simulink model "ampc_pH_lmpc"  (R2021a)
settings: Solver=VariableStepAuto  StartTime=0.0  StopTime=400  RelTol=1e-3
undefined symbols (not defined in the file or in its folder): sigbuilder_block
libraries: mpclib x1, simulink x1
settings Model: Creator=USER  LastModifiedBy=USER

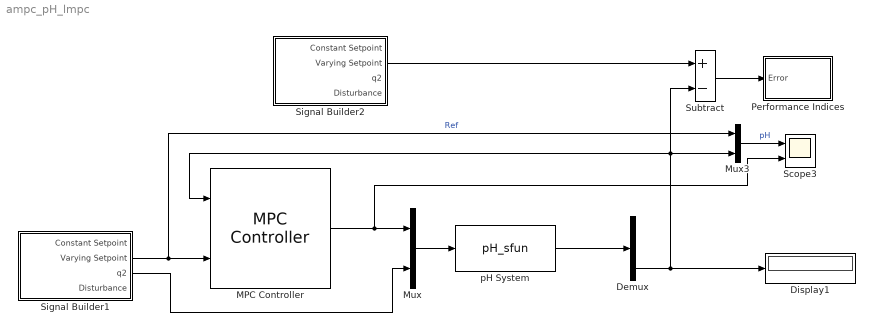
== system ampc_pH_lmpc ==
  Demux : Demux  Outputs=3
  Display1 : Display
  MPC Controller : mpclib/MPC Controller  SCDEnableBlockLinearizationSpecification=on  mpcobj=mpcobj_lmpc  is_multiple=0  enable_value=0  return_u0=off  updateMPCinCallerWorkspace=on  md_inport=off  mv_inport=off  uref_inport=off  return_cost=off  return_mvseq=off  return_qpstatus=off  return_xseq=off  return_state=off  return_ovseq=off  state_inport=off  umin_inport=off  umax_inport=off  ymin_inport=off  ymax_inport=off  cc_inport=off  ywt_inport=off  uwt_inport=off  duwt_inport=off  rhoeps_inport=off  pm_inport=off  MaximumP=10  HorizonChoice=FixedHorizon  n_ts=0.5  n_p=20  n_mv=1  n_md=0  n_ud=0  n_mo=1  n_uo=0  BlockDataType=double  SampleTimeInherited=off  switch_inport=off
  Mux : Mux  Inputs=2
  Mux3 : Mux  Inputs=2
  Performance Indices : Subsystem
  Scope3 : Scope  NumInputPorts=2
  Signal Builder1 : Subsystem  Tag=STV Subsys  LoadFcn=sigbuilder_block('load');  StartFcn=sigbuilder_block('start');  StopFcn=sigbuilder_block('stop');  ClipboardFcn=sigbuilder_block('clipboard');  mask(Sigbuilder block){tuvar=[0:10]}
      mask help: Simulink:masks:SigbuilderBlock_MD
      mask init:
      | if ~strcmp(get_param(bdroot(gcbh),'SimulationStatus'),'stopped') tuvar = sigbuilder_block('maskInit'); end
      settings: CopyFcn=sigbuilder_block('copy');  DeleteFcn=sigbuilder_block('delete');  ModelCloseFcn=sigbuilder_block('modelClose');  PreSaveFcn=sigbuilder_block('preSave');  PauseFcn=sigbuilder_block('pause');  ContinueFcn=sigbuilder_block('continue');  NameChangeFcn=sigbuilder_block('namechange');  OpenFcn=sigbuilder_block('open',[301 130.5 653.5 349.5 ]);  CloseFcn=sigbuilder_block('close');
      mask Display: plot(0, 0, 100, 100,[2, 2, 32, 32, 2], [68, 8, 8, 68, 68],[32, 2], [38, 38], [32, 19, 2],[53, 60, 44], [32, 17, 17, 2],[16, 16, 31, 31]);txt = getActiveGroup(gcbh);text(2, 100, txt,'verticalAlignment', 'top');
  Signal Builder2 : Subsystem  Tag=STV Subsys  LoadFcn=sigbuilder_block('load');  StartFcn=sigbuilder_block('start');  StopFcn=sigbuilder_block('stop');  ClipboardFcn=sigbuilder_block('clipboard');  mask(Sigbuilder block){tuvar=[0:10]}
      mask help: Simulink:masks:SigbuilderBlock_MD
      mask init:
      | if ~strcmp(get_param(bdroot(gcbh),'SimulationStatus'),'stopped') tuvar = sigbuilder_block('maskInit'); end
      settings: CopyFcn=sigbuilder_block('copy');  DeleteFcn=sigbuilder_block('delete');  ModelCloseFcn=sigbuilder_block('modelClose');  PreSaveFcn=sigbuilder_block('preSave');  PauseFcn=sigbuilder_block('pause');  ContinueFcn=sigbuilder_block('continue');  NameChangeFcn=sigbuilder_block('namechange');  OpenFcn=sigbuilder_block('open',[301 130.5 653.5 349.5 ]);  CloseFcn=sigbuilder_block('close');
      mask Display: plot(0, 0, 100, 100,[2, 2, 32, 32, 2], [68, 8, 8, 68, 68],[32, 2], [38, 38], [32, 19, 2],[53, 60, 44], [32, 17, 17, 2],[16, 16, 31, 31]);txt = getActiveGroup(gcbh);text(2, 100, txt,'verticalAlignment', 'top');
  Subtract : Sum  Inputs=+-
  pH System : S-Function  FunctionName=pH_sfun  SFunctionDeploymentMode=off  EnableBusSupport=off
  wires:
  Signal Builder1/2(Varying Setpoint) -> Mux3/1, MPC Controller/2  "Ref"
  Mux3/1 -> Scope3/1  "pH"
  Signal Builder2/2(Varying Setpoint) -> Subtract/1
  Subtract/1 -> Performance Indices/1(Error)
  MPC Controller/1 -> Scope3/2, Mux/1
  Signal Builder1/3(q2) -> Mux/2
  Demux/3 -> Display1/1, MPC Controller/1, Subtract/2, Mux3/2
  pH System/1 -> Demux/1
  Mux/1 -> pH System/1

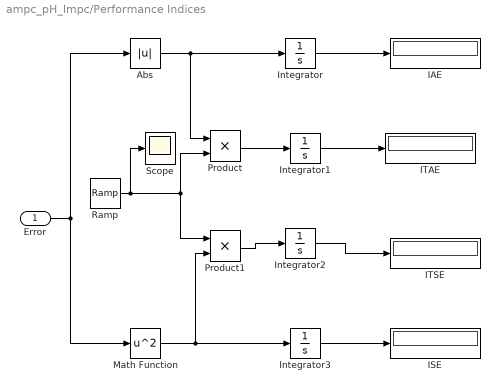
== system ampc_pH_lmpc/Performance Indices ==
  Error : Inport
  Abs : Abs
  IAE : Display
  ISE : Display
  ITAE : Display
  ITSE : Display
  Integrator{,1..3} (4 alike) : Integrator
  Math Function : Math  Operator=square  SignedPower=on  SaturateOnIntegerOverflow=on
  Product : Product  RndMeth=Zero
  Product1 : Product  RndMeth=Zero
  Ramp : simulink/Sources/Ramp  slope=1  start=0  InitialOutput=0
  Scope : Scope
  wires:
  Error/1 -> Math Function/1, Abs/1
  Abs/1 -> Integrator/1, Product/1
  Integrator/1 -> IAE/1
  Ramp/1 -> Product/2, Product1/1, Scope/1
  Math Function/1 -> Integrator3/1, Product1/2
  Product1/1 -> Integrator2/1
  Product/1 -> Integrator1/1
  Integrator3/1 -> ISE/1
  Integrator2/1 -> ITSE/1
  Integrator1/1 -> ITAE/1

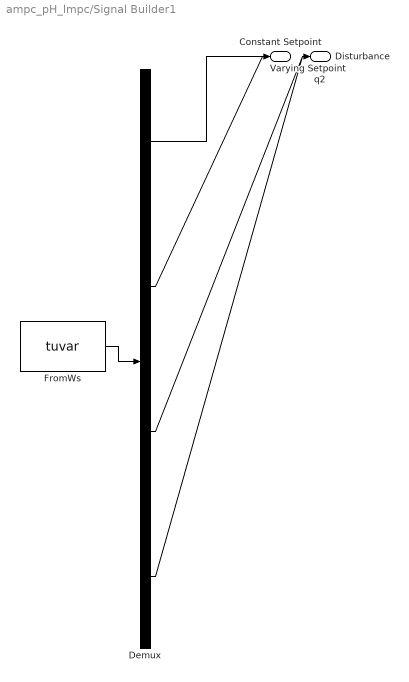
== system ampc_pH_lmpc/Signal Builder1 ==
  Demux : Demux  Tag=STV Demux
      settings: DisplayOption=none
  FromWs : FromWorkspace  Tag=STV FromWs  VariableName=tuvar
      SigBuilderData=|
      | common.afterFinalStr = 'Extrapolate'
      | common.sampleTime = 0
      | dataSet(1).timeRange = [0 400]
      | dataSet(1).name = 'Servo'
      | dataSet(2).timeRange = [0 400]
      | dataSet(2).name = 'Regulatory'
      | sbobj.Groups(1).Name = 'Servo'
      | sbobj.Groups(1).Signals(1).Name = 'Constant Setpoint'
      | sbobj.Groups(1).Signals(1).XData = [0 400]
      | sbobj.Groups(1).Signals(1).YData = [7 7]
      | sbobj.Groups(1).Signals(2).Name = 'Varying Setpoint'
      | sbobj.Groups(1).Signals(2).XData = [0 50 50 200 200 300 300 400]
      | sbobj.Groups(1).Signals(2).YData = [7 7 5 5 10 10 7 7]
      | sbobj.Groups(1).Signals(3).Name = 'q2'
      | sbobj.Groups(1).Signals(3).XData = [0 400]
      | sbobj.Groups(1).Signals(3).YData = [0.55 0.55]
      | sbobj.Groups(1).Signals(4).Name = 'Disturbance'
      | sbobj.Groups(1).Signals(4).XData = [0 100 100 200 200 300 300 400]
      | sbobj.Groups(1).Signals(4).YData = [0.55 0.55 1.5 1.5 0.05 0.05 0.55 0.55]
      | sbobj.Groups(1).TimeRange = [0 400]
      | sbobj.Groups(2).Name = 'Regulatory'
      | sbobj.Groups(2).Signals(1).Name = 'Constant Setpoint'
      | sbobj.Groups(2).Signals(1).XData = [0 400]
      | sbobj.Groups(2).Signals(1).YData = [0 0]
      | sbobj.Groups(2).Signals(2).Name = 'Varying Setpoint'
      | sbobj.Groups(2).Signals(2).XData = [0 400]
      | sbobj.Groups(2).Signals(2).YData = [7 7]
      | sbobj.Groups(2).Signals(3).Name = 'q2'
      | sbobj.Groups(2).Signals(3).XData = [0 30 30 60 60 90 90 120 120 150 150 400]
      | sbobj.Groups(2).Signals(3).YData = [0.55 0.55 1.2 1.2 2 2 1 1 0 0 0.55 0.55]
      | sbobj.Groups(2).Signals(4).Name = 'Disturbance'
      | sbobj.Groups(2).Signals(4).XData = [0 400]
      | sbobj.Groups(2).Signals(4).YData = [0 0]
      | sbobj.Groups(2).TimeRange = [0 400]
  Constant Setpoint : Outport  Tag=STV Outport
  Varying Setpoint : Outport  Tag=STV Outport  Port=2  VectorParamsAs1DForOutWhenUnconnected=off
  q2 : Outport  Tag=STV Outport  Port=3  VectorParamsAs1DForOutWhenUnconnected=off
  Disturbance : Outport  Tag=STV Outport  Port=4
  wires:
  FromWs/1 -> Demux/1
  Demux/1 -> Constant Setpoint/1
  Demux/2 -> Varying Setpoint/1
  Demux/3 -> q2/1
  Demux/4 -> Disturbance/1

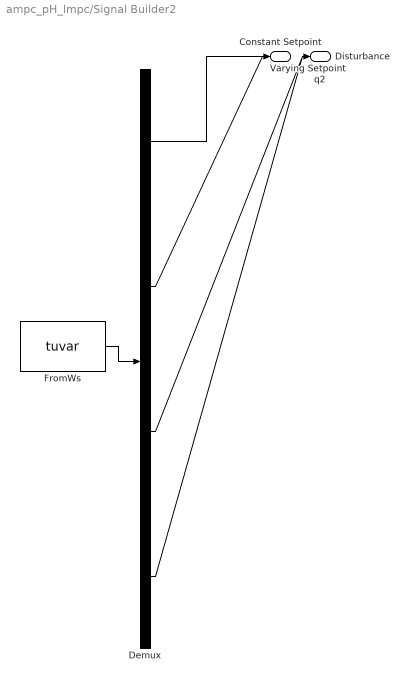
== system ampc_pH_lmpc/Signal Builder2 ==
  Demux : Demux  Tag=STV Demux
      settings: DisplayOption=none
  FromWs : FromWorkspace  Tag=STV FromWs  VariableName=tuvar
      SigBuilderData=|
      | common.afterFinalStr = 'Extrapolate'
      | common.sampleTime = 0
      | dataSet(1).timeRange = [0 400]
      | dataSet(1).name = 'Servo'
      | dataSet(2).timeRange = [0 400]
      | dataSet(2).name = 'Regulatory'
      | sbobj.Groups(1).Name = 'Servo'
      | sbobj.Groups(1).Signals(1).Name = 'Constant Setpoint'
      | sbobj.Groups(1).Signals(1).XData = [0 400]
      | sbobj.Groups(1).Signals(1).YData = [7 7]
      | sbobj.Groups(1).Signals(2).Name = 'Varying Setpoint'
      | sbobj.Groups(1).Signals(2).XData = [0 50 50 200 200 300 300 400]
      | sbobj.Groups(1).Signals(2).YData = [7 7 5 5 10 10 7 7]
      | sbobj.Groups(1).Signals(3).Name = 'q2'
      | sbobj.Groups(1).Signals(3).XData = [0 400]
      | sbobj.Groups(1).Signals(3).YData = [0.55 0.55]
      | sbobj.Groups(1).Signals(4).Name = 'Disturbance'
      | sbobj.Groups(1).Signals(4).XData = [0 100 100 200 200 300 300 400]
      | sbobj.Groups(1).Signals(4).YData = [0.55 0.55 1.5 1.5 0.05 0.05 0.55 0.55]
      | sbobj.Groups(1).TimeRange = [0 400]
      | sbobj.Groups(2).Name = 'Regulatory'
      | sbobj.Groups(2).Signals(1).Name = 'Constant Setpoint'
      | sbobj.Groups(2).Signals(1).XData = [0 400]
      | sbobj.Groups(2).Signals(1).YData = [0 0]
      | sbobj.Groups(2).Signals(2).Name = 'Varying Setpoint'
      | sbobj.Groups(2).Signals(2).XData = [0 400]
      | sbobj.Groups(2).Signals(2).YData = [7 7]
      | sbobj.Groups(2).Signals(3).Name = 'q2'
      | sbobj.Groups(2).Signals(3).XData = [0 30 30 60 60 90 90 120 120 150 150 400]
      | sbobj.Groups(2).Signals(3).YData = [0.55 0.55 1.2 1.2 2 2 1 1 0 0 0.55 0.55]
      | sbobj.Groups(2).Signals(4).Name = 'Disturbance'
      | sbobj.Groups(2).Signals(4).XData = [0 400]
      | sbobj.Groups(2).Signals(4).YData = [0 0]
      | sbobj.Groups(2).TimeRange = [0 400]
  Constant Setpoint : Outport  Tag=STV Outport
  Varying Setpoint : Outport  Tag=STV Outport  Port=2  VectorParamsAs1DForOutWhenUnconnected=off
  q2 : Outport  Tag=STV Outport  Port=3  VectorParamsAs1DForOutWhenUnconnected=off
  Disturbance : Outport  Tag=STV Outport  Port=4
  wires:
  FromWs/1 -> Demux/1
  Demux/1 -> Constant Setpoint/1
  Demux/2 -> Varying Setpoint/1
  Demux/3 -> q2/1
  Demux/4 -> Disturbance/1
